simulink model "Mask_Editor_Line_And_Sine_Wave"  (Simulink 10.0)
settings: Solver=VariableStepAuto  StartTime=0.0  StopTime=0.1  MaxStep=1e-3  RelTol=1e-3
libraries: simulink x1
settings Model: Creator=W002220B  LastModifiedBy=W002220B
settings DataIOCC: SaveFormat=Dataset  ReturnWorkspaceOutputs=on
settings OptimizationCC: LifeSpan=auto
settings DebuggingCC: UnderspecifiedInitializationDetection=Simplified  MergeDetectMultiDrivingBlocksExec=error  SFUnexpectedBacktrackingDiag=error  SFNoUnconditionalDefaultTransitionDiag=error  SFExecutionAtInitializationDiag=warning  ArithmeticOperatorsInVariantConditions=error
settings HardwareCC: ProdBitPerPointer=64  ProdBitPerSizeT=64  ProdBitPerPtrDiffT=64  ProdLargestAtomicFloat=Float  ProdIntDivRoundTo=Zero  ProdEndianess=LittleEndian  ProdWordSize=64  ProdHWDeviceType=Intel->x86-64 (Windows64)
settings ModelReferenceCC: PropagateSignalLabelsOutOfModel=on
settings SFSimCC: SimUseLocalCustomCode=on  CustomCodeUndefinedFunction=FilterOut
settings RTWCC: RTWUseLocalCustomCode=on
settings CodeAppCC: StateflowObjectComments=off
settings GRTTargetCC: TargetLangStandard=C99 (ISO)  CombineOutputUpdateFcns=on  GRTInterface=off
settings ConfigComp: CovMetricSettings=dwe  CovHtmlReporting=off  CovSaveCumulativeToWorkspaceVar=off  CovSaveSingleToWorkspaceVar=off

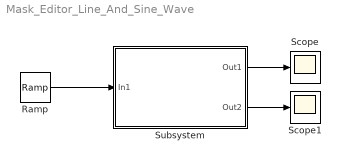
== system Mask_Editor_Line_And_Sine_Wave ==
  Ramp : simulink/Sources/Ramp  slope=10  start=0  InitialOutput=3
  Scope : Scope
  Scope1 : Scope
  Subsystem : Subsystem  mask{m=1, b=1, A=380, f=50}
      mask prompts: m "Slope"; b "Intercept"; A "SineAmplitude"; f "SineFreq"
      mask Display: image('C:\Users\W002220B\Desktop\IM_OLVC_run_hopeInsight.png'); % Use "Edit Image" on toolstrip to change.
  wires:
  Ramp/1 -> Subsystem/1(In1)
  Subsystem/1(Out1) -> Scope/1
  Subsystem/2(Out2) -> Scope1/1

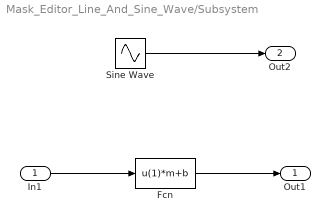
== system Mask_Editor_Line_And_Sine_Wave/Subsystem ==
  In1 : Inport
  Fcn : Fcn  Expr=u(1)*m+b
  Sine Wave : Sin  Amplitude=A  Frequency=2*pi*f  SampleTime=0
  Out1 : Outport
  Out2 : Outport  Port=2
  wires:
  In1/1 -> Fcn/1
  Fcn/1 -> Out1/1
  Sine Wave/1 -> Out2/1
